simulink model "lovely_chaos"  (Simulink 7.8)
settings: Solver=ode45  StartTime=0.0  StopTime=500.0  RelTol=1e-6
libraries: simulink x1
settings Model: Creator=Thanh  LastModifiedBy=Michael
settings DebuggingCC: FcnCallInpInsideContextMsg=Use local settings  StrictBusMsg=Warning

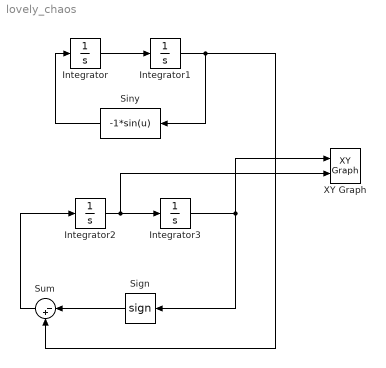
== system lovely_chaos ==
  Integrator : Integrator  InitialCondition=1.9
  Integrator1 : Integrator
  Integrator2 : Integrator
  Integrator3 : Integrator  InitialCondition=0.01
  Sign : Signum
  Siny : Fcn  Expr=-1*sin(u)
  Sum : Sum  Inputs=|-+
  XY Graph : simulink/Sinks/XY Graph  xmin=-25  xmax=25  ymin=-10  ymax=7  st=-1
  wires:
  Integrator/1 -> Integrator1/1
  Siny/1 -> Integrator/1
  Integrator1/1 -> Siny/1, Sum/2
  Integrator2/1 -> Integrator3/1, XY Graph/2
  Sign/1 -> Sum/1
  Integrator3/1 -> Sign/1, XY Graph/1
  Sum/1 -> Integrator2/1
